simulink model "tricycle_openloopcontrol"  (R2021a)
settings: Solver=VariableStepAuto  StartTime=0.0  StopTime=inf  RelTol=1e-3
libraries: simulink_extras x1, vehdynlibviscommon x1
settings Model: Creator=EGYPT  LastModifiedBy=Mostafa Ali
settings SolverCC: AlgebraicLoopSolver=TrustRegion
settings DebuggingCC: SFMachineParentedDataDiag=warning

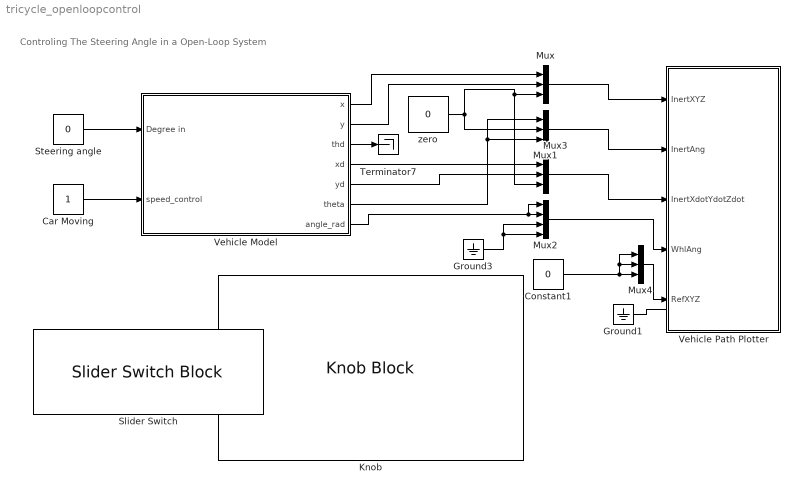
== system tricycle_openloopcontrol ==
  note: Controling The Steering Angle in a Open-Loop System
  "Car Moving " : Constant
  Constant1 : Constant  Value=0
  Ground1 : Ground
  Ground3 : Ground
  Knob : KnobBlock  ScaleMax=30
  Mux{,1,3..4} (4 alike) : Mux  Inputs=3
  Mux2 : Mux
  Slider Switch : SliderSwitchBlock
      settings: Values={{'Off', 'On'}, [0 1]}
  Steering angle : Constant  Value=0
  Terminator7 : Terminator
  "Vehicle Model " : Subsystem
      mask Display: image('D:\grad 1\matlab\maskKM.JPG'); % Use "Edit Image" on toolstrip to change.
  Vehicle Path Plotter : Subsystem  mask(Vehicle XY Plotter){extRef=on, extStats=off, extTireF=off, a=2, b=2, w=2, figBorder=10, bufferSize=1024, velNorm=5, tireFNorm=1000, pltDT=0.2}
      mask prompts: extRef "Plot path reference, extRef"; extStats "Display speed, RPM and Gear"; extTireF "Display tire forces"; a "Distance to front axle from CG, a [m]:"; b "Distance to rear axle from CG, b [m]:"; w "Track width, w [m]:"; figBorder "Distance to figure borders, figBorder [m]:"; bufferSize "Path buffer sampe size, bufferSize []:"; velNorm "Velocity vector scaling, velNorm [m*s/m]:"; tireFNorm "Tire force vector scaling, tireFNorm [m/N]:"; pltDT "Plot update rate, pltDT [s]:"
      mask help:
      | This block will display a MATLAB figure which indicates the vehicle path, current position and heading velocity.
      | An optional path reference is also provided.
      mask init:
      | block = gcb;
      | if autoblkschecksimstopped(block)
      |     ParamNames = {'extRef';'extStats';'extTireF';'extTireF'};
      |     PortNames = {'RefXYZ';'Stats';'TireFx';'TireFy'};
      |     for idx=1:length(PortNames)
      |         InportOption  = {'built-in/Ground', [PortNames{idx}, ' Ground'];...
      |             'built-in/Inport',PortNames{idx}};
      |         if ~strcmp(get_param(block,ParamNames{idx}),'on')
      |             NewBlkHdl = autoblksreplaceblock(block, InportOption, 1);
      |             set_param(NewBlkHdl, 'ShowName', 'off');
      |         else
      |             autoblksreplaceblock(block, InportOption, 2);
      |         end
      |     end
      |     InportNames = {'InertXYZ';'InertAng';'InertXdotYdotZdot';'WhlAng';'RefXYZ';'Stats';'TireFx';'TireFy'};
      |     FoundNames = get_param(find_system(block, 'LookUnderMasks', 'all', 'SearchDepth', 1, 'FollowLinks', 'on', 'BlockType', 'Inport'), 'Name');
      |     [~,PortI] = intersect(InportNames, FoundNames);
      |     PortI = sort(PortI);
      |     for idx = 1:length(PortI)
      |         set_param([block, '/', InportNames{PortI(idx)}], 'Port', num2str(idx));
      |     end
      | end
      mask TypeOptions a: Vehicle XY Plotter/a
      mask TypeOptions b: Vehicle XY Plotter/b
      mask TypeOptions w: Vehicle XY Plotter/w
      mask TypeOptions figBorder: Vehicle XY Plotter/figBorder
      mask TypeOptions bufferSize: Vehicle XY Plotter/bufferSize
      mask TypeOptions velNorm: Vehicle XY Plotter/velNorm
      mask TypeOptions tireFNorm: Vehicle XY Plotter/tireFNorm
      mask DialogControl Container3 Prompt: Plot and Display Options
  zero : Constant  Value=0
  wires:
  Steering angle/1 -> "Vehicle Model "/1(Degree in)
  "Car Moving "/1 -> "Vehicle Model "/2(speed_control)
  Mux/1 -> Vehicle Path Plotter/1(InertXYZ)
  Mux1/1 -> Vehicle Path Plotter/2(InertAng)
  Mux2/1 -> Vehicle Path Plotter/4(WhlAng)
  Mux3/1 -> Vehicle Path Plotter/3(InertXdotYdotZdot)
  Ground3/1 -> Mux2/3, Mux2/4
  "Vehicle Model "/1(x) -> Mux/1
  "Vehicle Model "/2(y) -> Mux/2
  zero/1 -> Mux1/2, Mux/3, Mux3/3
  "Vehicle Model "/4(xd) -> Mux3/1
  "Vehicle Model "/5(yd) -> Mux3/2
  Mux4/1 -> Vehicle Path Plotter/5(RefXYZ)
  Constant1/1 -> Mux4/1, Mux4/2, Mux4/3
  "Vehicle Model "/6(theta) -> Mux1/1, Mux1/3
  "Vehicle Model "/7(angle_rad) -> Mux2/1, Mux2/2
  Ground1/1 -> ?
  "Vehicle Model "/3(thd) -> Terminator7/1

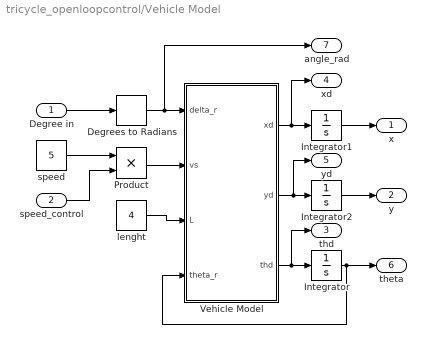
== system tricycle_openloopcontrol/Vehicle Model  ==
  Degree in : Inport
  speed_control : Inport  Port=2
  Degrees to Radians : simulink_extras/Transformations/Degrees to Radians
  Integrator : Integrator
  Integrator1 : Integrator
  Integrator2 : Integrator
  Product : Product
  "Vehicle Model " : MATLAB Function  TreatAsAtomicUnit=on
  lenght : Constant  Value=4
  speed : Constant  Value=5
  x : Outport
  y : Outport  Port=2
  thd : Outport  Port=3
  xd : Outport  Port=4
  yd : Outport  Port=5
  theta : Outport  Port=6
  angle_rad : Outport  Port=7
  wires:
  Integrator/1 -> "Vehicle Model "/4(theta_r), theta/1
  Degrees to Radians/1 -> angle_rad/1, "Vehicle Model "/1(delta_r)
  "Vehicle Model "/1(xd) -> xd/1, Integrator1/1
  Integrator2/1 -> y/1
  Product/1 -> "Vehicle Model "/2(vs)
  "Vehicle Model "/3(thd) -> Integrator/1, thd/1
  lenght/1 -> "Vehicle Model "/3(L)
  "Vehicle Model "/2(yd) -> Integrator2/1, yd/1
  speed/1 -> Product/1
  Degree in/1 -> Degrees to Radians/1
  Integrator1/1 -> x/1
  speed_control/1 -> Product/2

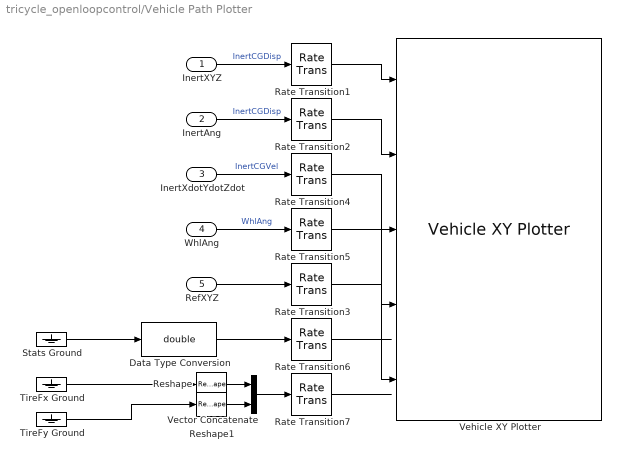
== system tricycle_openloopcontrol/Vehicle Path Plotter ==
  InertXYZ : Inport
  InertAng : Inport  Port=2
  InertXdotYdotZdot : Inport  Port=3
  WhlAng : Inport  Port=4
  RefXYZ : Inport  Port=5
  Data Type Conversion : DataTypeConversion  OutDataTypeStr=double
  Rate Transition{1..7} (7 alike) : RateTransition  Deterministic=off  OutPortSampleTime=pltDT
  Reshape : Reshape  OutputDimensionality=Row vector (2-D)
  Reshape1 : Reshape  OutputDimensionality=Row vector (2-D)
  Stats Ground : Ground
  TireFx Ground : Ground
  TireFy Ground : Ground
  Vector Concatenate : Concatenate  Mode=Multidimensional array
  Vehicle XY Plotter : vehdynlibviscommon/Vehicle XY Plotter  w=w  a=a  b=b  figBorder=figBorder  bufferSize=bufferSize  extStats=off  extTireF=off
      settings: SourceProductBaseCode=VE
  wires:
  Vector Concatenate/1 -> Rate Transition7/1
  Reshape1/1 -> Vector Concatenate/2
  Reshape/1 -> Vector Concatenate/1
  RefXYZ/1 -> Rate Transition3/1
  Rate Transition7/1 -> ?
  Data Type Conversion/1 -> Rate Transition6/1
  Rate Transition6/1 -> ?
  Rate Transition5/1 -> Vehicle XY Plotter/4
  Rate Transition4/1 -> Vehicle XY Plotter/3
  Rate Transition2/1 -> Vehicle XY Plotter/2
  Rate Transition1/1 -> Vehicle XY Plotter/1
  Rate Transition3/1 -> Vehicle XY Plotter/5
  WhlAng/1 -> Rate Transition5/1  "WhlAng"
  InertXYZ/1 -> Rate Transition1/1  "InertCGDisp"
  InertXdotYdotZdot/1 -> Rate Transition4/1  "InertCGVel"
  InertAng/1 -> Rate Transition2/1  "InertCGDisp"
  TireFx Ground/1 -> Reshape/1
  TireFy Ground/1 -> Reshape1/1
  Stats Ground/1 -> Data Type Conversion/1

== matlab function tricycle_openloopcontrol/Vehicle Model /Vehicle Model  ==
  data: delta_r input; xd output; yd output; thd output; vs input; L input; theta_r input
function[xd,yd,thd] = fcn(delta_r,vs,L,theta_r)
xd=vs*cos(delta_r)*cos(theta_r)
yd=vs*cos(delta_r)*sin(theta_r)
thd=(vs/L)*sin(delta_r)
